simulink model "imu"  (R2018b)
settings: Solver=FixedStepAuto  StartTime=0.0  StopTime=inf  FixedStep=0.01  RelTol=1e-3  EnableMultiTasking=on
libraries: arduinolib x6, simulink x1
settings Model: ExtModeTrigDuration=2  Creator=Filip  LastModifiedBy=Filip
settings OptimizationCC: EnhancedBackFolding=on  PassReuseOutputArgsAs=Individual arguments  MaxStackSize=64  OptimizeBlockOrder=speed  DifferentSizesBufferReuse=on  OptimizationCustomize=off
settings DebuggingCC: ParameterTunabilityLossMsg=error
settings HardwareCC: ProdBitPerInt=16  ProdBitPerPointer=16  ProdBitPerSizeT=16  ProdBitPerPtrDiffT=16  ProdLargestAtomicFloat=None  ProdWordSize=8  ProdHWDeviceType=Atmel->AVR
settings SFSimCC: MATLABDynamicMemAlloc=off
settings RTWCC: SystemTargetFile=ert.tlc  HardwareBoard=Arduino Nano 3.0  TemplateMakefile=ert_default_tmf  Toolchain=Arduino AVR  BuildConfiguration=Faster Runs  IncludeHyperlinkInReport=on
settings CodeAppCC: ForceParamTrailComments=on  IgnoreCustomStorageClasses=off  OperatorAnnotations=on  SimulinkDataObjDesc=on  SFDataObjDesc=on  InsertBlockDesc=on
settings ERTTargetCC: SupportContinuousTime=on  SupportVariableSizeSignals=on

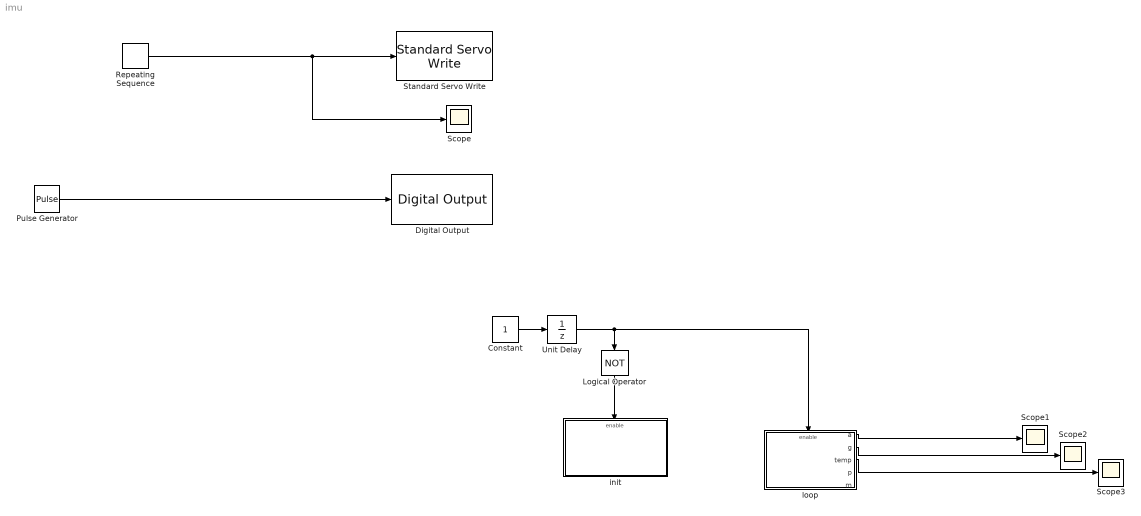
== system imu ==
  Constant : Constant  OutDataTypeStr=boolean  SampleTime=0.1
  Digital Output : arduinolib/Digital Output  pinNumber=13  blockPlatform=arduino
  Logical Operator : Logic  Operator=NOT  AllPortsSameDT=off  OutDataTypeStr=boolean
  Pulse Generator : DiscretePulseGenerator  PulseType=Time based  Period=1  PulseWidth=5
  Repeating Sequence : simulink/Sources/Repeating Sequence  rep_seq_t=[0 0.25 0.5]  rep_seq_y=[90-45 90+45 90-45]
  Scope{,1..3} (4 alike) : Scope
  Standard Servo Write : arduinolib/Standard Servo Write  pinNumber=2  ServoIndex=0  blockPlatform=ARDUINO
      settings: SourceProductName=Simulink Support Package for Arduino Hardware
  Unit Delay : UnitDelay  SampleTime=-1
  init : Subsystem
  loop : Subsystem
  wires:
  Pulse Generator/1 -> Digital Output/1
  Repeating Sequence/1 -> Scope/1, Standard Servo Write/1
  Constant/1 -> Unit Delay/1
  Logical Operator/1 -> init/Enable
  Unit Delay/1 -> loop/Enable, Logical Operator/1
  loop/1(a) -> Scope1/1
  loop/2(g) -> Scope2/1
  loop/3("temp ") -> Scope3/1

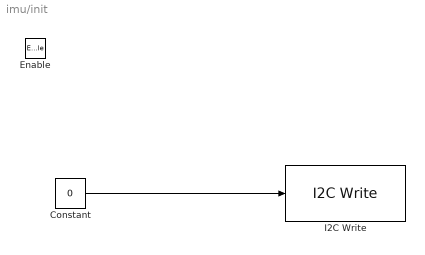
== system imu/init ==
  Enable : EnablePort
  Constant : Constant  Value=0
  I2C Write : arduinolib/I2C Write  I2CModule=0  Mode=Master  SlaveAddress=104  SlaveByteOrder=BigEndian  Direction=Transmitter  RegisterAddressMode=on  RegisterAddress=107  SlaveDataType=uint8  DataLength=1  NoAck=off  RepeatedStart=off  OutputStatus=off  blockPlatform=ARDUINO
      settings: SourceProductName=Simulink Support Package for Arduino Hardware  SourceProductBaseCode=ARDUINO
  wires:
  Constant/1 -> I2C Write/1

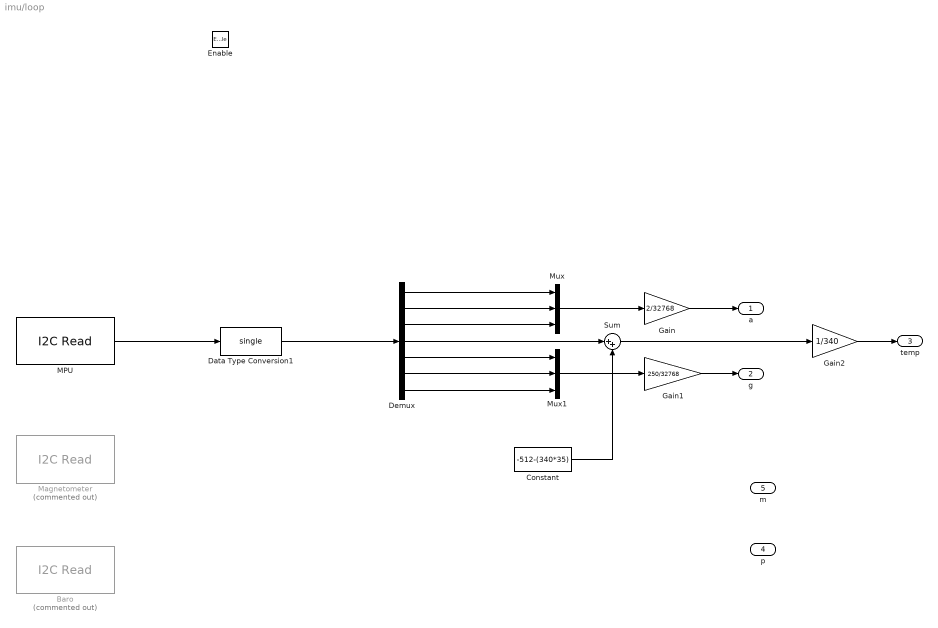
== system imu/loop ==
  Enable : EnablePort
  Baro : arduinolib/I2C Read  Commented=on  I2CModule=0  Mode=Master  SlaveAddress=hex2dec('77')  SlaveByteOrder=BigEndian  Direction=Receiver  RegisterAddressMode=on  RegisterAddress=59  SlaveDataType=int16  DataLength=7  NoAck=off  RepeatedStart=off  OutputStatus=off  blockPlatform=ARDUINO  SampleTime=0.1
      settings: SourceProductName=Simulink Support Package for Arduino Hardware  SourceProductBaseCode=ARDUINO
  Constant : Constant  Value=-512-(340*35)
  Data Type Conversion1 : DataTypeConversion  OutDataTypeStr=single
  Demux : Demux  Outputs=7
  Gain : Gain  Gain=2/32768
  Gain1 : Gain  Gain=250/32768
  Gain2 : Gain  Gain=1/340
  MPU : arduinolib/I2C Read  I2CModule=0  Mode=Master  SlaveAddress=hex2dec('68')  SlaveByteOrder=BigEndian  Direction=Receiver  RegisterAddressMode=on  RegisterAddress=hex2dec('3B')  SlaveDataType=int16  DataLength=7  NoAck=off  RepeatedStart=off  OutputStatus=off  blockPlatform=ARDUINO  SampleTime=0.1
      settings: SourceProductName=Simulink Support Package for Arduino Hardware  SourceProductBaseCode=ARDUINO
  Magnetometer : arduinolib/I2C Read  Commented=on  I2CModule=0  Mode=Master  SlaveAddress=hex2dec('1E')  SlaveByteOrder=BigEndian  Direction=Receiver  RegisterAddressMode=on  RegisterAddress=59  SlaveDataType=int16  DataLength=7  NoAck=off  RepeatedStart=off  OutputStatus=off  blockPlatform=ARDUINO  SampleTime=0.1
      settings: SourceProductName=Simulink Support Package for Arduino Hardware  SourceProductBaseCode=ARDUINO
  Mux : Mux  Inputs=3
  Mux1 : Mux  Inputs=3
  Sum : Sum  Inputs=|++
  a : Outport
  g : Outport  Port=2
  "temp " : Outport  Port=3
  p : Outport  Port=4
  m : Outport  Port=5
  wires:
  Gain/1 -> a/1
  MPU/1 -> Data Type Conversion1/1
  Data Type Conversion1/1 -> Demux/1
  Demux/1 -> Mux/1
  Demux/2 -> Mux/2
  Demux/3 -> Mux/3
  Demux/5 -> Mux1/1
  Demux/6 -> Mux1/2
  Demux/7 -> Mux1/3
  Mux/1 -> Gain/1
  Mux1/1 -> Gain1/1
  Gain1/1 -> g/1
  Gain2/1 -> "temp "/1
  Demux/4 -> Sum/1
  Sum/1 -> Gain2/1
  Constant/1 -> Sum/2
